simulink model "passive_suspension"  (R2020a)
settings: Solver=VariableStepAuto  StartTime=0.0  StopTime=10.0  RelTol=1e-3
settings Model: Creator=USER  LastModifiedBy=USER

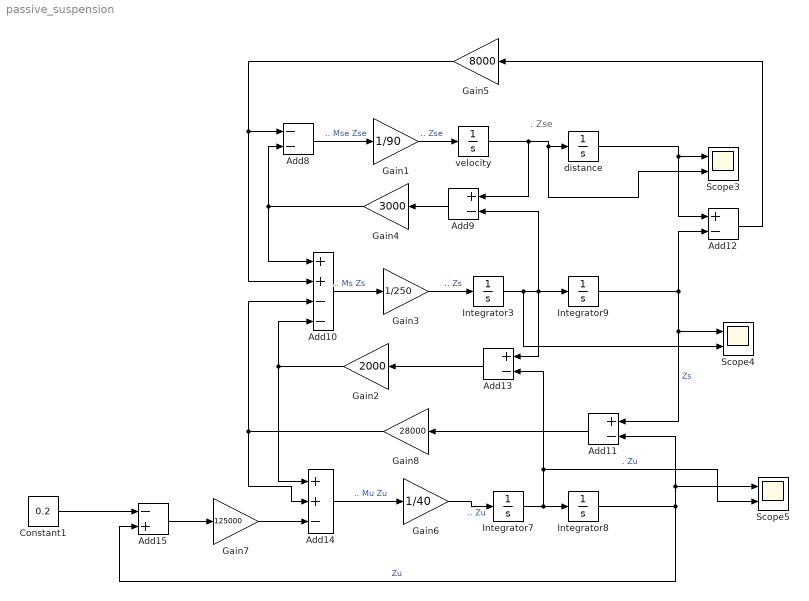
== system passive_suspension ==
  note: .
      | Zse
  Add10 : Sum  Inputs=++--
  Add{9,11..13} (4 alike) : Sum  Inputs=+-
  Add14 : Sum  Inputs=++-
  Add15 : Sum  Inputs=-+
  Add8 : Sum  Inputs=--
  Constant1 : Constant  Value=0.2
  Gain1 : Gain  Gain=1/90
  Gain2 : Gain  Gain=2000
  Gain3 : Gain  Gain=1/250
  Gain4 : Gain  Gain=3000
  Gain5 : Gain  Gain=8000
  Gain6 : Gain  Gain=1/40
  Gain7 : Gain  Gain=125000
  Gain8 : Gain  Gain=28000
  Integrator{3,7..9} (4 alike) : Integrator
  Scope3 : Scope  NumInputPorts=2
  Scope4 : Scope  NumInputPorts=2
  Scope5 : Scope  NumInputPorts=2
  distance : Integrator
  velocity : Integrator
  wires:
  Gain5/1 -> Add10/2, Add8/1
  Add8/1 -> Gain1/1  ".. Mse Zse"
  Integrator8/1 -> Add15/2, Add11/2, Scope5/1  "Zu"
  Gain4/1 -> Add10/1, Add8/2
  Add13/1 -> Gain2/1
  Integrator7/1 -> Add13/2, Scope5/2, Integrator8/1  ". Zu"
  Gain6/1 -> Integrator7/1  ".. Zu"
  Add14/1 -> Gain6/1  ".. Mu Zu"
  Gain2/1 -> Add14/1, Add10/4
  Add9/1 -> Gain4/1
  Integrator3/1 -> Scope4/2, Integrator9/1, Add13/1, Add9/2
  Gain1/1 -> velocity/1  ".. Zse"
  distance/1 -> Add12/1, Scope3/1
  velocity/1 -> Add9/1, distance/1, Scope3/2
  Add10/1 -> Gain3/1  ".. Ms Zs"
  Add12/1 -> Gain5/1
  Integrator9/1 -> Add11/1, Scope4/1, Add12/2  "Zs"
  Constant1/1 -> Add15/1
  Gain8/1 -> Add14/2, Add10/3
  Add15/1 -> Gain7/1
  Add11/1 -> Gain8/1
  Gain3/1 -> Integrator3/1  ".. Zs"
  Gain7/1 -> Add14/3
